simulink model "inverted_pendulum"  (R2023b)
settings: Solver=VariableStepAuto  StartTime=0.0  StopTime=10  RelTol=1e-3
values from neighbouring files (symbols this model uses):
  A = [0   1 ... (first row only)    [DC_motor_example_LQR_v2.m]    (also in inverted_pendulum_main.m = [ 0         0               1                   0)
  B = [0 ... (first row only)    [DC_motor_example_LQR_v2.m]    (also in inverted_pendulum_main.m = [       0)
  Cc = eye(4)    [inverted_pendulum_main.m]
  Dc = zeros(4, 1)    [inverted_pendulum_main.m]
  K = lqr(A,B,Q,R)    [DC_motor_example_LQR_v2.m]    (also in inverted_pendulum_main.m = lqr(sys, Qf, Rf))
settings Model: PauseTimes=20  Creator=loicdewit  LastModifiedBy=loicdewit

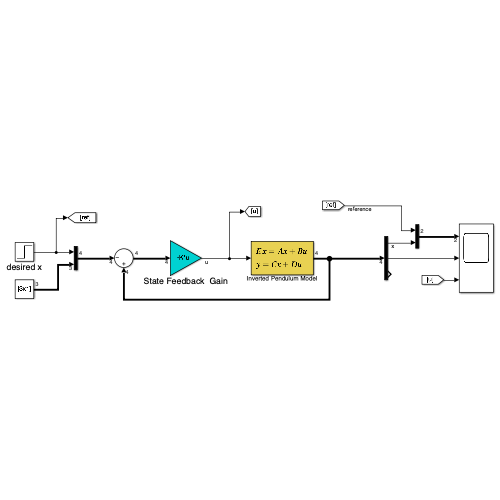
[thumbnail: Simulink's stored preview of the top-level diagram]
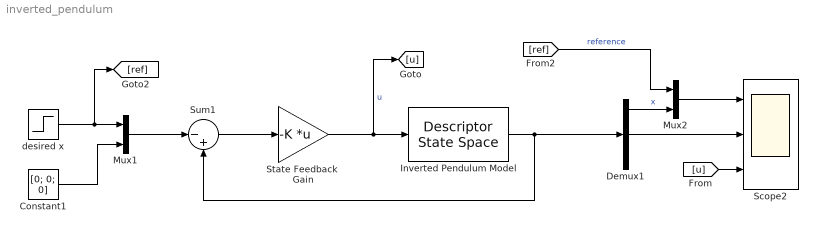
== system inverted_pendulum ==
  Constant1 : Constant  Value=[0; 0; 0]
  Demux1 : Demux  Outputs=[1 1 2]
  Inverted Pendulum Model : DescriptorStateSpace  E=eye(4)  A=A  B=B  C=Cc  D=Dc
  Mux1 : Mux  Inputs=2
  Mux2 : Mux  Inputs=2
  Scope2 : Scope  NumInputPorts=3
  State Feedback  Gain : Gain  Gain=-K  Multiplication=Matrix(K*u)
  Sum1 : Sum  Inputs=|-+
  desired x : Step  SampleTime=0
  wires:
  Inverted Pendulum Model/1 -> Sum1/2, Demux1/1
  State Feedback  Gain/1 -> [u], Inverted Pendulum Model/1  "u"
  Constant1/1 -> Mux1/2
  desired x/1 -> [ref], Mux1/1
  Mux1/1 -> Sum1/1
  Sum1/1 -> State Feedback  Gain/1
  Demux1/1 -> Mux2/2  "x"
  [u] -> Scope2/3
  Mux2/1 -> Scope2/1
  Demux1/2 -> Scope2/2
  [ref] -> Mux2/1  "reference"
